simulink model "Control_Unit_Software_Case1"  (R2018b)
settings: Solver=FixedStepAuto  StartTime=0.0  StopTime=4  RelTol=1e-3
values from neighbouring files (symbols this model uses):
  A = [-(bm*(n^2) + bg)/(Jm*(n^2) + Jg) Kt*n/(Jm*(n^2) + Jg) ... (first row only)    [acceptatieTestScript.m]
  B = [0 ... (first row only)    [acceptatieTestScript.m]
  C = [1 0]    [acceptatieTestScript.m]
  D = [0]    [acceptatieTestScript.m]
  Kdi = dlqr(Ad,Bd,Q,R)    [acceptatieTestScript.m]
  n = 16.5    [acceptatieTestScript.m]
  Tsc = 1/20000    (= 5e-05)    [acceptatieTestScript.m]
undefined symbols (not defined in the file or in its folder): DiscIntNeverNeededParam, sigbuilder_block
libraries: dspswit3 x29, simulink x14, powerlib_meascontrol x6, dspsigops x4, pePwmGenerator x4, peLuenbergerObserver x2, peGeneralControl x1
(part 2 of 2)

== system Control_Unit_Software_Case1/Beveiliging/Temperatuur vertraging Links ==
  Timer : Inport
  Input : Inport  Port=2
  Counter2 : dspswit3/Counter  Direction=Up  CountEvent=Rising edge  CounterSize=User defined  MaxCount=300  InitialCount=0  Output=Hit  HitValue=300  ResetInput=on  SamplesPerFrame=1  Ts=1  CntDtype=double  HitDtype=Logical
  Edge Detector : dspswit3/Edge Detector  InputProcessing=Columns as channels (frame based)
      settings: SourceProductName=DSP System Toolbox  SourceProductBaseCode=DS
  Edge Detector Rise/Fall : Subsystem
  OR1 : Logic  Operator=OR  IconShape=distinctive  AllPortsSameDT=off  OutDataTypeStr=boolean
  Sample and Hold : dspsigops/Sample and Hold  trig=Rising edge  initCond=0  latchinput=off
  Scope : Scope
  Scope1 : Scope
  Output : Outport
  wires:
  Timer/1 -> Counter2/1
  Sample and Hold/1 -> Output/1
  OR1/1 -> Edge Detector/1
  Edge Detector/1 -> Scope1/1, Sample and Hold/Trigger
  Counter2/1 -> OR1/1
  Input/1 -> Scope/1, OR1/2, Sample and Hold/1, Edge Detector Rise/Fall/1(In)
  Edge Detector Rise/Fall/1(Out) -> Counter2/2

== system Control_Unit_Software_Case1/Beveiliging/Temperatuur vertraging Rechts  ==
  Timer : Inport
  Input : Inport  Port=2
  Counter2 : dspswit3/Counter  Direction=Up  CountEvent=Rising edge  CounterSize=User defined  MaxCount=300  InitialCount=0  Output=Hit  HitValue=300  ResetInput=on  SamplesPerFrame=1  Ts=1  CntDtype=double  HitDtype=Logical
  Edge Detector : dspswit3/Edge Detector  InputProcessing=Columns as channels (frame based)
      settings: SourceProductName=DSP System Toolbox  SourceProductBaseCode=DS
  Edge Detector Rise/Fall : Subsystem
  OR1 : Logic  Operator=OR  IconShape=distinctive  AllPortsSameDT=off  OutDataTypeStr=boolean
  Sample and Hold : dspsigops/Sample and Hold  trig=Rising edge  initCond=0  latchinput=off
  Scope : Scope
  Scope1 : Scope
  Output : Outport
  wires:
  Timer/1 -> Counter2/1
  Sample and Hold/1 -> Output/1
  OR1/1 -> Edge Detector/1
  Edge Detector/1 -> Scope1/1, Sample and Hold/Trigger
  Counter2/1 -> OR1/1
  Input/1 -> Scope/1, OR1/2, Sample and Hold/1, Edge Detector Rise/Fall/1(In)
  Edge Detector Rise/Fall/1(Out) -> Counter2/2

== system Control_Unit_Software_Case1/Stuurhoek Converter/Output > 100% ==
  L_In : Inport
  R_In : Inport  Port=2
  Compare To Constant : simulink/Logic and Bit Operations/Compare To Constant  relop=>  const=1  OutDataTypeStr=boolean
  Compare To Constant1 : simulink/Logic and Bit Operations/Compare To Constant  relop=>  const=1  OutDataTypeStr=boolean
  Divide4 : Product  Inputs=**
  Divide5 : Product  Inputs=**
  Subtract : Sum  Inputs=+-
  Subtract1 : Sum  Inputs=-+
  L_Out : Outport
  R_Out : Outport  Port=2
  wires:
  Compare To Constant1/1 -> Subtract1/1, Divide4/1
  Compare To Constant/1 -> Subtract/2, Divide5/2
  Subtract1/1 -> Divide4/2
  Subtract/1 -> Divide5/1
  L_In/1 -> Subtract/1, Compare To Constant/1
  Divide5/1 -> R_Out/1
  R_In/1 -> Subtract1/2, Compare To Constant1/1
  Divide4/1 -> L_Out/1

== system Control_Unit_Software_Case1/Beveiliging/Stroom vertraging Links/Edge Detector Rise//Fall ==
  In : Inport
  Edge Detector1 : dspswit3/Edge Detector  InputProcessing=Columns as channels (frame based)
      settings: SourceProductName=DSP System Toolbox  SourceProductBaseCode=DS
  Edge Detector2 : dspswit3/Edge Detector  InputProcessing=Columns as channels (frame based)
      settings: SourceProductName=DSP System Toolbox  SourceProductBaseCode=DS
  NOT : Logic  Operator=NOT  IconShape=distinctive  AllPortsSameDT=off  OutDataTypeStr=boolean
  OR : Logic  Operator=OR  IconShape=distinctive  AllPortsSameDT=off  OutDataTypeStr=boolean
  Out : Outport
  wires:
  In/1 -> NOT/1, Edge Detector1/1
  NOT/1 -> Edge Detector2/1
  Edge Detector1/1 -> OR/1
  OR/1 -> Out/1
  Edge Detector2/1 -> OR/2

== system Control_Unit_Software_Case1/Beveiliging/Stroom vertraging Rechts/Edge Detector Rise//Fall ==
  In : Inport
  Edge Detector1 : dspswit3/Edge Detector  InputProcessing=Columns as channels (frame based)
      settings: SourceProductName=DSP System Toolbox  SourceProductBaseCode=DS
  Edge Detector2 : dspswit3/Edge Detector  InputProcessing=Columns as channels (frame based)
      settings: SourceProductName=DSP System Toolbox  SourceProductBaseCode=DS
  NOT : Logic  Operator=NOT  IconShape=distinctive  AllPortsSameDT=off  OutDataTypeStr=boolean
  OR : Logic  Operator=OR  IconShape=distinctive  AllPortsSameDT=off  OutDataTypeStr=boolean
  Out : Outport
  wires:
  In/1 -> NOT/1, Edge Detector1/1
  NOT/1 -> Edge Detector2/1
  Edge Detector1/1 -> OR/1
  OR/1 -> Out/1
  Edge Detector2/1 -> OR/2

== system Control_Unit_Software_Case1/Beveiliging/Temperatuur vertraging Links/Edge Detector Rise//Fall ==
  In : Inport
  Edge Detector1 : dspswit3/Edge Detector  InputProcessing=Columns as channels (frame based)
      settings: SourceProductName=DSP System Toolbox  SourceProductBaseCode=DS
  Edge Detector2 : dspswit3/Edge Detector  InputProcessing=Columns as channels (frame based)
      settings: SourceProductName=DSP System Toolbox  SourceProductBaseCode=DS
  NOT : Logic  Operator=NOT  IconShape=distinctive  AllPortsSameDT=off  OutDataTypeStr=boolean
  OR : Logic  Operator=OR  IconShape=distinctive  AllPortsSameDT=off  OutDataTypeStr=boolean
  Out : Outport
  wires:
  In/1 -> NOT/1, Edge Detector1/1
  NOT/1 -> Edge Detector2/1
  Edge Detector1/1 -> OR/1
  OR/1 -> Out/1
  Edge Detector2/1 -> OR/2

== system Control_Unit_Software_Case1/Beveiliging/Temperatuur vertraging Rechts /Edge Detector Rise//Fall ==
  In : Inport
  Edge Detector1 : dspswit3/Edge Detector  InputProcessing=Columns as channels (frame based)
      settings: SourceProductName=DSP System Toolbox  SourceProductBaseCode=DS
  Edge Detector2 : dspswit3/Edge Detector  InputProcessing=Columns as channels (frame based)
      settings: SourceProductName=DSP System Toolbox  SourceProductBaseCode=DS
  NOT : Logic  Operator=NOT  IconShape=distinctive  AllPortsSameDT=off  OutDataTypeStr=boolean
  OR : Logic  Operator=OR  IconShape=distinctive  AllPortsSameDT=off  OutDataTypeStr=boolean
  Out : Outport
  wires:
  In/1 -> NOT/1, Edge Detector1/1
  NOT/1 -> Edge Detector2/1
  Edge Detector1/1 -> OR/1
  OR/1 -> Out/1
  Edge Detector2/1 -> OR/2

== matlab function Control_Unit_Software_Case1/Snelheidsmeter/Periode meting ==
  data: speedPulse input; pulses output; speedPulseBuf data_store_memory; pulseCount data_store_memory; period input; i data_store_memory; fs input; j data_store_memory; reset input
function pulses = fcn(speedPulse,period, fs, reset)

global pulseCount;
global speedPulseBuf;
global i;
global j;

if reset == 1
    speedPulseBuf = uint8(zeros(size(speedPulseBuf)));
end

bufTime = period*fs + 1;

if i > bufTime
    i = uint32(1);
end

if j > bufTime
    j = uint32(1);
end

speedPulseBuf(i) = speedPulse;
pulseCount = pulseCount + uint32(speedPulse);
pulseCount = pulseCount - uint32(speedPulseBuf(j));

i = i + 1;
j = j + 1;

pulses = pulseCount;

== matlab function Control_Unit_Software_Case1/Snelheidsmeter1/Periode meting ==
  data: speedPulse input; pulses output; speedPulseBuf data_store_memory; pulseCount data_store_memory; period input; i data_store_memory; fs input; j data_store_memory; reset input
function pulses = fcn(speedPulse,period, fs, reset)

global pulseCount;
global speedPulseBuf;
global i;
global j;

if reset == 1
    speedPulseBuf = uint8(zeros(size(speedPulseBuf)));
end

bufTime = period*fs + 1;

if i > bufTime
    i = uint32(1);
end

if j > bufTime
    j = uint32(1);
end

speedPulseBuf(i) = speedPulse;
pulseCount = pulseCount + uint32(speedPulse);
pulseCount = pulseCount - uint32(speedPulseBuf(j));

i = i + 1;
j = j + 1;

pulses = pulseCount;
